simulink model "CanalMultiTrajets"  (Simulink 10.1)
settings: Solver=VariableStepAuto  StartTime=0.0  StopTime=2e6/9e6  RelTol=1e-3
undefined symbols (not defined in the file or in its folder): doppler
libraries: commchan3 x4, commrandsrc3 x1, commdigbbndam3 x1
settings Model: Creator=iba  LastModifiedBy=iba
settings DataIOCC: SaveFormat=Dataset  ReturnWorkspaceOutputs=on
settings OptimizationCC: LifeSpan=auto
settings DebuggingCC: UnderspecifiedInitializationDetection=Simplified  MergeDetectMultiDrivingBlocksExec=error  SFUnexpectedBacktrackingDiag=error  SFNoUnconditionalDefaultTransitionDiag=error  SFExecutionAtInitializationDiag=warning  ArithmeticOperatorsInVariantConditions=error
settings HardwareCC: ProdBitPerPointer=64  ProdBitPerSizeT=64  ProdBitPerPtrDiffT=64  ProdLargestAtomicFloat=Float  ProdIntDivRoundTo=Zero  ProdEndianess=LittleEndian  ProdWordSize=64  ProdHWDeviceType=Intel->x86-64 (Windows64)
settings ModelReferenceCC: PropagateSignalLabelsOutOfModel=on
settings SFSimCC: SimUseLocalCustomCode=on  CustomCodeUndefinedFunction=FilterOut
settings RTWCC: RTWUseLocalCustomCode=on
settings CodeAppCC: StateflowObjectComments=off
settings GRTTargetCC: TargetLangStandard=C99 (ISO)  CombineOutputUpdateFcns=on  GRTInterface=off
settings ConfigComp: CovMetricSettings=dwe  CovHtmlReporting=off  CovSaveCumulativeToWorkspaceVar=off  CovSaveSingleToWorkspaceVar=off  CovExternalEMLEnable=on

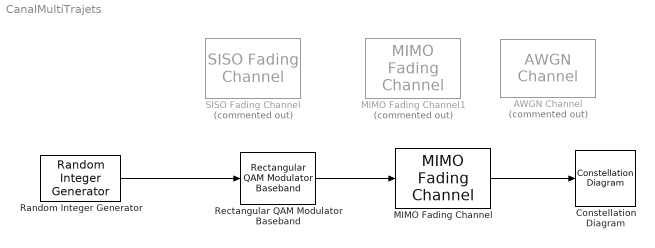
== system CanalMultiTrajets ==
  AWGN Channel : commchan3/AWGN Channel  Commented=on  InputProcessing=Columns as channels (frame based)  seed=67  noiseMode="Signal to noise ratio  (Eb/No)"  EbNodB=10  EsNodB=10  SNRdB=10  bitsPerSym=1  Ps=1  Tsym=1  variance=1
  Constellation Diagram : ConstellationDiagram
  MIMO Fading Channel : commchan3/MIMO Fading Channel  InheritSampleRate=on  SampleRate=1  PathDelays=0  AveragePathGains=0  NormalizePathGains=on  FadingDistribution=Rayleigh  KFactor=3  DirectPathDopplerShift=0  DirectPathInitialPhase=0  MaximumDopplerShift=0.001  DopplerSpectrum=doppler('Jakes')  SpatialCorrelationSpecification=Separate Tx Rx  SpatialCorrelationMatrix=[1 0 0 0; 0 1 0 0; 0 0 1 0; 0 0 0 1]  NumTransmitAntennas=2  NumReceiveAntennas=2  TransmitCorrelationMatrix=[1 0; 0 1]  ReceiveCorrelationMatrix=[1 0; 0 1]  AntennaSelection=Off  NormalizeChannelOutputs=on  SimulateUsing=Interpreted execution  FadingTechnique=Filtered Gaussian noise  NumSinusoids=48  InitialTimeSource=Property  InitialTime=0  RandomStream=mt19937ar with seed  Seed=73  PathGainsOutputPort=off  Visualization=Off  AntennaPairsToDisplay=[ 1, 1 ]  PathsForDopplerDisplay=1  SamplesToDisplay=25%
      settings: SourceProductBaseCode=CM
  MIMO Fading Channel1 : commchan3/MIMO Fading Channel  Commented=on  InheritSampleRate=on  SampleRate=1  PathDelays=0  AveragePathGains=0  NormalizePathGains=on  FadingDistribution=Rayleigh  KFactor=3  DirectPathDopplerShift=0  DirectPathInitialPhase=0  MaximumDopplerShift=0.001  DopplerSpectrum=doppler('Jakes')  SpatialCorrelationSpecification=None  SpatialCorrelationMatrix=[1 0 0 0; 0 1 0 0; 0 0 1 0; 0 0 0 1]  NumTransmitAntennas=2  NumReceiveAntennas=2  TransmitCorrelationMatrix=[1 0; 0 1]  ReceiveCorrelationMatrix=[1 0; 0 1]  AntennaSelection=Off  NormalizeChannelOutputs=on  SimulateUsing=Interpreted execution  FadingTechnique=Filtered Gaussian noise  NumSinusoids=48  InitialTimeSource=Property  InitialTime=0  RandomStream=mt19937ar with seed  Seed=73  PathGainsOutputPort=off  Visualization=Off  AntennaPairsToDisplay=[ 1, 1 ]  PathsForDopplerDisplay=1  SamplesToDisplay=25%
      settings: SourceProductBaseCode=CM
  Random Integer Generator : commrandsrc3/Random Integer Generator  SetSize=4  SeedSource=Parameter  Seed=37  SampleTime=1/9e6  SamplesPerFrame=1000  OutputDataType=double  SimulateUsing=Interpreted execution
  Rectangular QAM Modulator Baseband : commdigbbndam3/Rectangular QAM Modulator Baseband  M=4  InType=Integer  Enc=Gray  Mapping=[0:15]  PowType=Min. distance between symbols  MinDist=2  AvgPow=1  PeakPow=1  Ph=0  outDtype=double  outWordLen=16  outUDDataType=sfix(16)  outFracLenMode=Best precision  outFracLen=15  outDataTypeStr=double  outLastDataTypeStr=double
  SISO Fading Channel : commchan3/SISO Fading Channel  Commented=on  InheritSampleRate=on  SampleRate=1  PathDelays=0  AveragePathGains=0  NormalizePathGains=on  FadingDistribution=Rayleigh  KFactor=3  DirectPathDopplerShift=0  DirectPathInitialPhase=0  MaximumDopplerShift=0.001  DopplerSpectrum=doppler('Jakes')  RandomStream=mt19937ar with seed  Seed=73  PathGainsOutputPort=off  ChannelFilterDelayOutputPort=off  SimulateUsing=Interpreted execution  Visualization=Off  PathsForDopplerDisplay=1  SamplesToDisplay=25%
  wires:
  Random Integer Generator/1 -> Rectangular QAM Modulator Baseband/1
  MIMO Fading Channel/1 -> Constellation Diagram/1
  Rectangular QAM Modulator Baseband/1 -> MIMO Fading Channel/1
